simulink model "BSD_VehicleSignal_SWC"  (R2024a)
settings: Solver=FixedStepDiscrete  StartTime=0.0  StopTime=10.0  FixedStep=0.02  RelTol=1e-3
libraries: simulink x2
settings Model: Creator=pc  LastModifiedBy=pc
settings OptimizationCC: DefaultParameterBehavior=Inlined  EnhancedBackFolding=on  PassReuseOutputArgsAs=Individual arguments  ZeroExternalMemoryAtStartup=off  ZeroInternalMemoryAtStartup=off  OptimizeBlockOrder=speed  DifferentSizesBufferReuse=on  OptimizationCustomize=off  EfficientTunableParamExpr=on
settings DebuggingCC: ParameterTunabilityLossMsg=error
settings SFSimCC: MATLABDynamicMemAlloc=off
settings RTWCC: Description=AUTOSAR  SystemTargetFile=autosar.tlc  GenCodeOnly=on  PackageGeneratedCodeAndArtifacts=on  TemplateMakefile=ert_default_tmf  GenerateReport=on  Toolchain=MinGW64 | CMake/gmake (64-bit Windows)  BuildConfiguration=Release  LaunchReport=on  DataTypeReplacement=CDataTypesFixedWidth  CheckMdlBeforeBuild=Warning
settings CodeAppCC: ForceParamTrailComments=on  IgnoreCustomStorageClasses=off  OperatorAnnotations=on  SimulinkDataObjDesc=on  SFDataObjDesc=on  InsertBlockDesc=on
settings STFCustomTargetCC: MultiwordLength=256  ParMdlRefBuildCompliant=on  CompOptLevelCompliant=on  IncludeMdlTerminateFcn=off  CombineOutputUpdateFcns=on  SuppressErrorStatus=on  ERTCustomFileBanners=on  SupportNonFinite=off  SupportComplex=off  SupportContinuousTime=off  SupportNonInlinedSFcns=off  RemoveResetFunc=on  MATLABClassNameForMDSCustomization=Simulink.SoftwareTarget.ERTCustomization  AutosarCompliant=on  GRTInterface=off  LookupTableObjectStructAxisOrder=2,1,3,4,...  LUTObjectStructOrderEvenSpacing=Size,Table,Breakpoints  SystemTargetFile=autosar.tlc
settings ERTTargetCC: TargetLangStandard=C99 (ISO)  ConcurrentExecutionCompliant=off  IncludeMdlTerminateFcn=off  SuppressErrorStatus=on  SupportNonFinite=off  SupportComplex=off  ModelStepFunctionPrototypeControlCompliant=off  CPPClassGenCompliant=off  AutosarCompliant=on  LookupTableObjectStructAxisOrder=2,1,3,4,...  LUTObjectStructOrderEvenSpacing=Size,Table,Breakpoints  InlinedParameterPlacement=NonHierarchical  ERTCustomFileTemplate=example_file_process.tlc  BooleanTrueId=TRUE  BooleanFalseId=FALSE

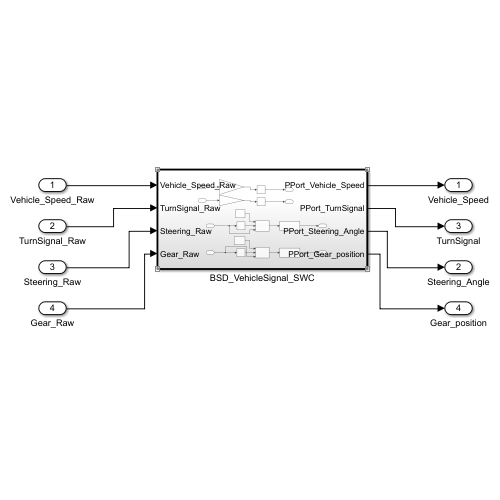
[thumbnail: Simulink's stored preview of the top-level diagram]
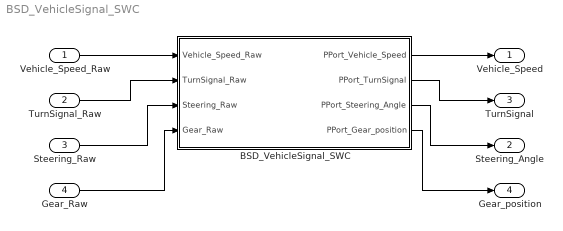
== system BSD_VehicleSignal_SWC ==
  Vehicle_Speed_Raw : Inport  OutDataTypeStr=uint16
  TurnSignal_Raw : Inport  Port=2  OutDataTypeStr=uint8
  Steering_Raw : Inport  Port=3  OutDataTypeStr=int16
  Gear_Raw : Inport  Port=4  OutDataTypeStr=uint8
  BSD_VehicleSignal_SWC : Subsystem  TreatAsAtomicUnit=on  SystemSampleTime=0.02
  Vehicle_Speed : Outport  OutDataTypeStr=single
  Steering_Angle : Outport  Port=2  OutDataTypeStr=single
  TurnSignal : Outport  Port=3  OutDataTypeStr=uint8
  Gear_position : Outport  Port=4  OutDataTypeStr=uint8
  wires:
  Steering_Raw/1 -> BSD_VehicleSignal_SWC/3(Steering_Raw)
  TurnSignal_Raw/1 -> BSD_VehicleSignal_SWC/2(TurnSignal_Raw)
  Vehicle_Speed_Raw/1 -> BSD_VehicleSignal_SWC/1(Vehicle_Speed_Raw)
  BSD_VehicleSignal_SWC/1(PPort_Vehicle_Speed) -> Vehicle_Speed/1
  Gear_Raw/1 -> BSD_VehicleSignal_SWC/4(Gear_Raw)
  BSD_VehicleSignal_SWC/4(PPort_Gear_position) -> Gear_position/1
  BSD_VehicleSignal_SWC/3(PPort_Steering_Angle) -> Steering_Angle/1
  BSD_VehicleSignal_SWC/2(PPort_TurnSignal) -> TurnSignal/1

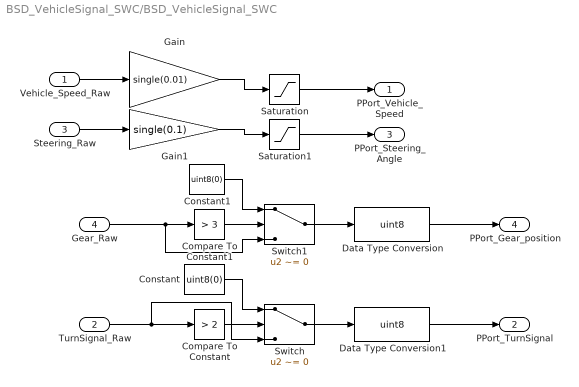
== system BSD_VehicleSignal_SWC/BSD_VehicleSignal_SWC ==
  Vehicle_Speed_Raw : Inport  OutDataTypeStr=uint16
  TurnSignal_Raw : Inport  Port=2
  Steering_Raw : Inport  Port=3  OutDataTypeStr=int16
  Gear_Raw : Inport  Port=4
  Compare To Constant : simulink/Logic and Bit Operations/Compare To Constant  relop=>  const=2  OutDataTypeStr=uint8
  Compare To Constant1 : simulink/Logic and Bit Operations/Compare To Constant  relop=>  const=3  OutDataTypeStr=uint8
  Constant : Constant  Value=uint8(0)  OutDataTypeStr=uint8
  Constant1 : Constant  Value=uint8(0)  OutDataTypeStr=uint8
  Data Type Conversion : DataTypeConversion  OutDataTypeStr=uint8  SaturateOnIntegerOverflow=off  RndMeth=Floor
  Data Type Conversion1 : DataTypeConversion  OutDataTypeStr=uint8  SaturateOnIntegerOverflow=off  RndMeth=Floor
  Gain : Gain  Gain=single(0.01)  OutDataTypeStr=single
  Gain1 : Gain  Gain=single(0.1)  OutDataTypeStr=single
  Saturation : Saturate  UpperLimit=300  LowerLimit=0  OutDataTypeStr=single
  Saturation1 : Saturate  UpperLimit=900  LowerLimit=-900  OutDataTypeStr=single
  Switch : Switch  Criteria=u2 ~= 0  OutDataTypeStr=uint8  SaturateOnIntegerOverflow=off  InputSameDT=off
  Switch1 : Switch  Criteria=u2 ~= 0  OutDataTypeStr=uint8  SaturateOnIntegerOverflow=off  InputSameDT=off
  PPort_Vehicle_Speed : Outport  OutDataTypeStr=single
  PPort_TurnSignal : Outport  Port=2  OutDataTypeStr=uint8
  PPort_Steering_Angle : Outport  Port=3  OutDataTypeStr=single
  PPort_Gear_position : Outport  Port=4  OutDataTypeStr=uint8
  wires:
  TurnSignal_Raw/1 -> Switch/3, Compare To Constant/1
  Gear_Raw/1 -> Switch1/3, Compare To Constant1/1
  Steering_Raw/1 -> Gain1/1
  Vehicle_Speed_Raw/1 -> Gain/1
  Compare To Constant1/1 -> Switch1/2
  Constant1/1 -> Switch1/1
  Constant/1 -> Switch/1
  Gain1/1 -> Saturation1/1
  Gain/1 -> Saturation/1
  Compare To Constant/1 -> Switch/2
  Saturation/1 -> PPort_Vehicle_Speed/1
  Saturation1/1 -> PPort_Steering_Angle/1
  Switch1/1 -> Data Type Conversion/1
  Data Type Conversion/1 -> PPort_Gear_position/1
  Switch/1 -> Data Type Conversion1/1
  Data Type Conversion1/1 -> PPort_TurnSignal/1
